simulink model "TBRe19_ECU_1_DAY1_EDIT_190719"  (R2017b)
settings: Solver=FixedStepDiscrete  StartTime=0.0  StopTime=inf  FixedStep=0.0001  RelTol=1e-3
PostLoadFcn:
  | model_init();
libraries: simulink x17
(part 3 of 6)

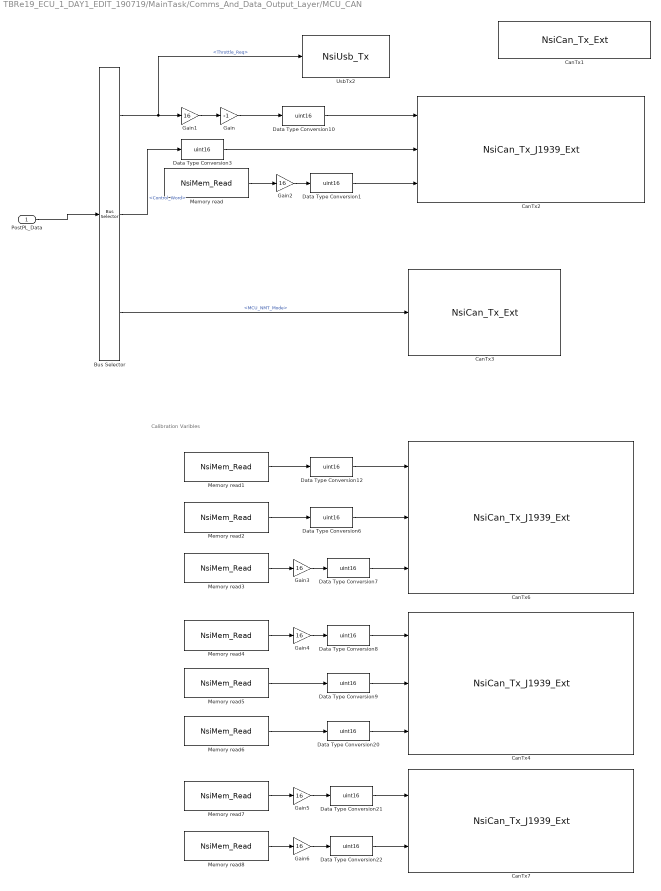
== system TBRe19_ECU_1_DAY1_EDIT_190719/MainTask/Comms_And_Data_Output_Layer/MCU_CAN ==
  note: Calibration Varibles
  PostPL_Data : Inport
  Bus Selector : BusSelector  OutputSignals=VFL_Data.Drive_Data.Throttle_Req,VFL_Data.VOM_Data.Control_Word,VFL_Data.VOM_Data.MCU_NMT_Mode
  CanTx1 : S-Function  FunctionName=NsiCan_Tx_Ext  Parameters=data_can,channel,msg_name,ident,ident_type,dlc,signals,is_physical,is_canfd,is_crc  SFunctionDeploymentMode=off  EnableBusSupport=off  mask(MUXlink Can Tx){data_can=1;HIGH_SPEED;500Kbps;No;C:\Users\TBRe-admin\Documents\Database\TBRe19_DBC_190617.dbc;0;;;0;HIGH_SPEED;500Kbps;120 Ohm;C:\Users\TBRe-admin\Documents\Database\TBRe19_DBC_190517.dbc;0;;;0;HIGH_SPEED;1000Kbps;120 Ohm;D:\TOOLS\MUXLINK\R2011b\MUXlink\misc\BASE_CAN_MUXLAB4.dbc;0;;;0;HIGH_SPEED;500Kbps;120 Ohm;D:\TOOLS\MUXLINK\R2011b\MUXlink\misc\j1939_adapt.dbc;0;;;0;HIGH_SPEED;1000Kbps;No;D:\TOOLS\MUXLINK\R2011b\MUXlink\misc\BASE_CAN_MUXLAB4.dbc;0;;, channel=1, msg_name=MCU_Sync_MSG, ident=0x080, ident_type=STD, dlc=0, signals=, is_physical=0, is_canfd=0, is_crc=0}
      mask prompts: data_can "data can"; msg_name "msg name"
      mask help: Transmit a frame on a CAN Channel.
      mask init:
      | NsiCan_Tx_Ext_InitializationFcn();
      settings: OpenFcn=NsiCan_Tx_Ext_OpenFcn();
      mask Help:
      | eval('block=get_param(gcb, ''RTWdata'');')
      | web([docroot '\toolbox\MUXlink\html\blocks/' block.MUXlink_BlockType '.html'])
      mask Callback data_can: NsiCan_Tx_Ext_ApplyFcn(1);
      mask Callback channel: NsiCan_Tx_Ext_ApplyFcn(2);
      mask Callback msg_name: NsiCan_Tx_Ext_ApplyFcn(3);
      mask Callback ident: NsiCan_Tx_Ext_ApplyFcn(4);
      mask Callback ident_type: NsiCan_Tx_Ext_ApplyFcn(5);
      mask Callback dlc: NsiCan_Tx_Ext_ApplyFcn(6);
      mask Callback signals: NsiCan_Tx_Ext_ApplyFcn(7);
      mask Callback is_physical: NsiCan_Tx_Ext_ApplyFcn(7);
      mask Callback is_canfd: NsiCan_Tx_Ext_ApplyFcn(7);
      mask Callback is_crc: NsiCan_Tx_Ext_ApplyFcn(7);
      mask Display: image(imread('nsi.bmp'));text(0.5, 0.3, 'TX_MCU_Sync_MSG_CAN1', 'horizontalAlignment', 'center', 'verticalAlignment', 'base');plot([0.05 0.05 0.05 0.05 0.05 0.05 0.05 0.05 0.05 0.05]);
  CanTx2 : S-Function  FunctionName=NsiCan_Tx_J1939_Ext  Parameters=data_can,channel,msg_name,ident,ident_type,dlc,signals,is_SA_Masked,is_physical,is_canfd  SFunctionDeploymentMode=off  EnableBusSupport=off  mask(MUXlink Can Tx){data_can=1;HIGH_SPEED;500Kbps;No;C:\Users\Peter\Google_Drive\Year_5\TBRe\03-Design_Files\ECU\ECU-Model\TBRe19_DBC.dbc;0;;;0;HIGH_SPEED;500Kbps;120 Ohm;C:\Users\TBRe-admin\Documents\Database\TBRe19_DBC_190517.dbc;0;;;0;HIGH_SPEED;1000Kbps;120 Ohm;D:\TOOLS\MUXLINK\R2011b\MUXlink\misc\BASE_CAN_MUXLAB4.dbc;0;;;0;HIGH_SPEED;500Kbps;120 Ohm;D:\TOOLS\MUXLINK\R2011b\MUXlink\misc\j1939_adapt.dbc;0;;;0;HIGH_SPEED;1000Kbps;No;D:\TOOLS\MUXLINK\R2011b\MUXlink\misc\BASE_CAN_MUXLAB4.dbc;0;;, channel=1, msg_name=HC1_Demands, ident=0x19107171, ident_type=XTD, dlc=8, signals=Torque_Request;1;0;-16;0.062500;0.000000;Nm;ControlWord;1;16;-16;1.000000;0.000000;_;Torque_Traction_Limit;1;32;-16;0.062500;0.000000;Nm, is_SA_Masked=1, is_physical=0, is_canfd=0}
      mask prompts: data_can "data can"; msg_name "msg name"
      mask help: Transmit a frame on a CAN Channel.
      mask init:
      | NsiCan_Tx_J1939_Ext_InitializationFcn();
      settings: OpenFcn=NsiCan_Tx_J1939_Ext_OpenFcn();
      mask Help:
      | eval('block=get_param(gcb, ''RTWdata'');')
      | web([docroot '\toolbox\MUXlink\html\blocks/' block.MUXlink_BlockType '.html'])
      mask Callback data_can: NsiCan_Tx_J1939_Ext_ApplyFcn(1);
      mask Callback channel: NsiCan_Tx_J1939_Ext_ApplyFcn(2);
      mask Callback msg_name: NsiCan_Tx_J1939_Ext_ApplyFcn(3);
      mask Callback ident: NsiCan_Tx_J1939_Ext_ApplyFcn(4);
      mask Callback ident_type: NsiCan_Tx_J1939_Ext_ApplyFcn(5);
      mask Callback dlc: NsiCan_Tx_J1939_Ext_ApplyFcn(6);
      mask Callback signals: NsiCan_Tx_J1939_Ext_ApplyFcn(7);
      mask Callback is_SA_Masked: NsiCan_Tx_J1939_Ext_ApplyFcn(8);
      mask Callback is_physical: NsiCan_Tx_J1939_Ext_ApplyFcn(9)
      mask Callback is_canfd: NsiCan_Tx_J1939_Ext_ApplyFcn(10)
      mask Display: image(imread('nsi.bmp'));text(0.5, 0.3, 'J1939_PGN  HC1_Demandschannel CAN1', 'horizontalAlignment', 'center', 'verticalAlignment', 'base');plot([0.05 0.05 0.05 0.05 0.05 0.05 0.05 0.05 0.05 0.05]); port_label('input',1, 'Torque_Request'); port_label('input',2, 'ControlWord'); port_label('input',3, 'Torque_Traction_Limit');
  CanTx3 : S-Function  FunctionName=NsiCan_Tx_Ext  Parameters=data_can,channel,msg_name,ident,ident_type,dlc,signals,is_physical,is_canfd,is_crc  SFunctionDeploymentMode=off  EnableBusSupport=off  mask(MUXlink Can Tx){data_can=1;HIGH_SPEED;500Kbps;No;C:\Users\TBRe-admin\Documents\TBReVCU\TBRe19_DBC.dbc;0;;;0;HIGH_SPEED;500Kbps;120 Ohm;C:\Users\TBRe-admin\Documents\Database\TBRe19_DBC_190517.dbc;0;;;0;HIGH_SPEED;1000Kbps;120 Ohm;D:\TOOLS\MUXLINK\R2011b\MUXlink\misc\BASE_CAN_MUXLAB4.dbc;0;;;0;HIGH_SPEED;500Kbps;120 Ohm;D:\TOOLS\MUXLINK\R2011b\MUXlink\misc\j1939_adapt.dbc;0;;;0;HIGH_SPEED;1000Kbps;No;D:\TOOLS\MUXLINK\R2011b\MUXlink\misc\BASE_CAN_MUXLAB4.dbc;0;;, channel=1, msg_name=MCU_NMT_Broadcast, ident=0x070, ident_type=STD, dlc=2, signals=NMT_Command;1;0;8;1.000000;0.000000;_, is_physical=1, is_canfd=0, is_crc=0}
      mask prompts: data_can "data can"; msg_name "msg name"
      mask help: Transmit a frame on a CAN Channel.
      mask init:
      | NsiCan_Tx_Ext_InitializationFcn();
      settings: OpenFcn=NsiCan_Tx_Ext_OpenFcn();
      mask Help:
      | eval('block=get_param(gcb, ''RTWdata'');')
      | web([docroot '\toolbox\MUXlink\html\blocks/' block.MUXlink_BlockType '.html'])
      mask Callback data_can: NsiCan_Tx_Ext_ApplyFcn(1);
      mask Callback channel: NsiCan_Tx_Ext_ApplyFcn(2);
      mask Callback msg_name: NsiCan_Tx_Ext_ApplyFcn(3);
      mask Callback ident: NsiCan_Tx_Ext_ApplyFcn(4);
      mask Callback ident_type: NsiCan_Tx_Ext_ApplyFcn(5);
      mask Callback dlc: NsiCan_Tx_Ext_ApplyFcn(6);
      mask Callback signals: NsiCan_Tx_Ext_ApplyFcn(7);
      mask Callback is_physical: NsiCan_Tx_Ext_ApplyFcn(7);
      mask Callback is_canfd: NsiCan_Tx_Ext_ApplyFcn(7);
      mask Callback is_crc: NsiCan_Tx_Ext_ApplyFcn(7);
      mask Display: image(imread('nsi.bmp'));text(0.5, 0.1, 'TX_MCU_NMT_Broadcast_CAN1', 'horizontalAlignment', 'center', 'verticalAlignment', 'base');plot([0.05 0.05 0.05 0.05 0.05 0.05 0.05 0.05 0.05 0.05]); port_label('input',1, 'NMT_Command');
  CanTx4 : S-Function  FunctionName=NsiCan_Tx_J1939_Ext  Parameters=data_can,channel,msg_name,ident,ident_type,dlc,signals,is_SA_Masked,is_physical,is_canfd  SFunctionDeploymentMode=off  EnableBusSupport=off  mask(MUXlink Can Tx){data_can=1;HIGH_SPEED;500Kbps;No;C:\Users\Peter\Google_Drive\Year_5\TBRe\03-Design_Files\ECU\ECU-Model\TBRe19_DBC.dbc;0;;;0;HIGH_SPEED;500Kbps;120 Ohm;C:\Users\TBRe-admin\Documents\Database\TBRe19_DBC_190517.dbc;0;;;0;HIGH_SPEED;1000Kbps;120 Ohm;D:\TOOLS\MUXLINK\R2011b\MUXlink\misc\BASE_CAN_MUXLAB4.dbc;0;;;0;HIGH_SPEED;500Kbps;120 Ohm;D:\TOOLS\MUXLINK\R2011b\MUXlink\misc\j1939_adapt.dbc;0;;;0;HIGH_SPEED;1000Kbps;No;D:\TOOLS\MUXLINK\R2011b\MUXlink\misc\BASE_CAN_MUXLAB4.dbc;0;;, channel=1, msg_name=HC3_Battery_Demands, ident=0x19127171, ident_type=XTD, dlc=8, signals=DC_Link_Voltage_Target;1;32;-16;0.062500;0.000000;V;DC_Link_Imax_Recharge;1;16;-16;1.000000;0.000000;A;DC_Link_Imax_Discharge;1;0;-16;1.000000;0.000000;A, is_SA_Masked=1, is_physical=0, is_canfd=0}
      mask prompts: data_can "data can"; msg_name "msg name"
      mask help: Transmit a frame on a CAN Channel.
      mask init:
      | NsiCan_Tx_J1939_Ext_InitializationFcn();
      settings: OpenFcn=NsiCan_Tx_J1939_Ext_OpenFcn();
      mask Help:
      | eval('block=get_param(gcb, ''RTWdata'');')
      | web([docroot '\toolbox\MUXlink\html\blocks/' block.MUXlink_BlockType '.html'])
      mask Callback data_can: NsiCan_Tx_J1939_Ext_ApplyFcn(1);
      mask Callback channel: NsiCan_Tx_J1939_Ext_ApplyFcn(2);
      mask Callback msg_name: NsiCan_Tx_J1939_Ext_ApplyFcn(3);
      mask Callback ident: NsiCan_Tx_J1939_Ext_ApplyFcn(4);
      mask Callback ident_type: NsiCan_Tx_J1939_Ext_ApplyFcn(5);
      mask Callback dlc: NsiCan_Tx_J1939_Ext_ApplyFcn(6);
      mask Callback signals: NsiCan_Tx_J1939_Ext_ApplyFcn(7);
      mask Callback is_SA_Masked: NsiCan_Tx_J1939_Ext_ApplyFcn(8);
      mask Callback is_physical: NsiCan_Tx_J1939_Ext_ApplyFcn(9)
      mask Callback is_canfd: NsiCan_Tx_J1939_Ext_ApplyFcn(10)
      mask Display: image(imread('nsi.bmp'));text(0.5, 0.3, 'J1939_PGN  HC3_Battery_Demandschannel CAN1', 'horizontalAlignment', 'center', 'verticalAlignment', 'base');plot([0.05 0.05 0.05 0.05 0.05 0.05 0.05 0.05 0.05 0.05]); port_label('input',1, 'DC_Link_Voltage_Target'); port_label('input',2, 'DC_Link_Imax_Recharge'); port_label('input',3, 'DC_Link_Imax_Discharge');
  CanTx6 : S-Function  FunctionName=NsiCan_Tx_J1939_Ext  Parameters=data_can,channel,msg_name,ident,ident_type,dlc,signals,is_SA_Masked,is_physical,is_canfd  SFunctionDeploymentMode=off  EnableBusSupport=off  mask(MUXlink Can Tx){data_can=1;HIGH_SPEED;500Kbps;No;C:\Users\Peter\Google_Drive\Year_5\TBRe\03-Design_Files\ECU\ECU-Model\TBRe19_DBC.dbc;0;;;0;HIGH_SPEED;500Kbps;120 Ohm;C:\Users\TBRe-admin\Documents\Database\TBRe19_DBC_190517.dbc;0;;;0;HIGH_SPEED;1000Kbps;120 Ohm;D:\TOOLS\MUXLINK\R2011b\MUXlink\misc\BASE_CAN_MUXLAB4.dbc;0;;;0;HIGH_SPEED;500Kbps;120 Ohm;D:\TOOLS\MUXLINK\R2011b\MUXlink\misc\j1939_adapt.dbc;0;;;0;HIGH_SPEED;1000Kbps;No;D:\TOOLS\MUXLINK\R2011b\MUXlink\misc\BASE_CAN_MUXLAB4.dbc;0;;, channel=1, msg_name=HC2_Demands, ident=0x19117171, ident_type=XTD, dlc=8, signals=Speed_Limit_Reverse;1;32;-16;1.000000;0.000000;RPM;Speed_Limit_Forward;1;16;-16;1.000000;0.000000;RPM;Torque_Regen_Limit;1;0;-16;0.062500;0.000000;_, is_SA_Masked=1, is_physical=0, is_canfd=0}
      mask prompts: data_can "data can"; msg_name "msg name"
      mask help: Transmit a frame on a CAN Channel.
      mask init:
      | NsiCan_Tx_J1939_Ext_InitializationFcn();
      settings: OpenFcn=NsiCan_Tx_J1939_Ext_OpenFcn();
      mask Help:
      | eval('block=get_param(gcb, ''RTWdata'');')
      | web([docroot '\toolbox\MUXlink\html\blocks/' block.MUXlink_BlockType '.html'])
      mask Callback data_can: NsiCan_Tx_J1939_Ext_ApplyFcn(1);
      mask Callback channel: NsiCan_Tx_J1939_Ext_ApplyFcn(2);
      mask Callback msg_name: NsiCan_Tx_J1939_Ext_ApplyFcn(3);
      mask Callback ident: NsiCan_Tx_J1939_Ext_ApplyFcn(4);
      mask Callback ident_type: NsiCan_Tx_J1939_Ext_ApplyFcn(5);
      mask Callback dlc: NsiCan_Tx_J1939_Ext_ApplyFcn(6);
      mask Callback signals: NsiCan_Tx_J1939_Ext_ApplyFcn(7);
      mask Callback is_SA_Masked: NsiCan_Tx_J1939_Ext_ApplyFcn(8);
      mask Callback is_physical: NsiCan_Tx_J1939_Ext_ApplyFcn(9)
      mask Callback is_canfd: NsiCan_Tx_J1939_Ext_ApplyFcn(10)
      mask Display: image(imread('nsi.bmp'));text(0.5, 0.3, 'J1939_PGN  HC2_Demandschannel CAN1', 'horizontalAlignment', 'center', 'verticalAlignment', 'base');plot([0.05 0.05 0.05 0.05 0.05 0.05 0.05 0.05 0.05 0.05]); port_label('input',1, 'Speed_Limit_Reverse'); port_label('input',2, 'Speed_Limit_Forward'); port_label('input',3, 'Torque_Regen_Limit');
  CanTx7 : S-Function  FunctionName=NsiCan_Tx_J1939_Ext  Parameters=data_can,channel,msg_name,ident,ident_type,dlc,signals,is_SA_Masked,is_physical,is_canfd  SFunctionDeploymentMode=off  EnableBusSupport=off  mask(MUXlink Can Tx){data_can=1;HIGH_SPEED;500Kbps;No;C:\Users\Peter\Google_Drive\Year_5\TBRe\03-Design_Files\ECU\ECU-Model\TBRe19_DBC.dbc;0;;;0;HIGH_SPEED;500Kbps;120 Ohm;C:\Users\TBRe-admin\Documents\Database\TBRe19_DBC_190517.dbc;0;;;0;HIGH_SPEED;1000Kbps;120 Ohm;D:\TOOLS\MUXLINK\R2011b\MUXlink\misc\BASE_CAN_MUXLAB4.dbc;0;;;0;HIGH_SPEED;500Kbps;120 Ohm;D:\TOOLS\MUXLINK\R2011b\MUXlink\misc\j1939_adapt.dbc;0;;;0;HIGH_SPEED;1000Kbps;No;D:\TOOLS\MUXLINK\R2011b\MUXlink\misc\BASE_CAN_MUXLAB4.dbc;0;;, channel=1, msg_name=HC4_Debug_Demands, ident=0x19137171, ident_type=XTD, dlc=8, signals=Debug_Id_direct_control;1;16;-16;0.062500;0.000000;A;Debug_Iq_direct_control;1;0;-16;0.062500;0.000000;A, is_SA_Masked=1, is_physical=0, is_canfd=0}
      mask prompts: data_can "data can"; msg_name "msg name"
      mask help: Transmit a frame on a CAN Channel.
      mask init:
      | NsiCan_Tx_J1939_Ext_InitializationFcn();
      settings: OpenFcn=NsiCan_Tx_J1939_Ext_OpenFcn();
      mask Help:
      | eval('block=get_param(gcb, ''RTWdata'');')
      | web([docroot '\toolbox\MUXlink\html\blocks/' block.MUXlink_BlockType '.html'])
      mask Callback data_can: NsiCan_Tx_J1939_Ext_ApplyFcn(1);
      mask Callback channel: NsiCan_Tx_J1939_Ext_ApplyFcn(2);
      mask Callback msg_name: NsiCan_Tx_J1939_Ext_ApplyFcn(3);
      mask Callback ident: NsiCan_Tx_J1939_Ext_ApplyFcn(4);
      mask Callback ident_type: NsiCan_Tx_J1939_Ext_ApplyFcn(5);
      mask Callback dlc: NsiCan_Tx_J1939_Ext_ApplyFcn(6);
      mask Callback signals: NsiCan_Tx_J1939_Ext_ApplyFcn(7);
      mask Callback is_SA_Masked: NsiCan_Tx_J1939_Ext_ApplyFcn(8);
      mask Callback is_physical: NsiCan_Tx_J1939_Ext_ApplyFcn(9)
      mask Callback is_canfd: NsiCan_Tx_J1939_Ext_ApplyFcn(10)
      mask Display: image(imread('nsi.bmp'));text(0.5, 0.3, 'J1939_PGN  HC4_Debug_Demandschannel CAN1', 'horizontalAlignment', 'center', 'verticalAlignment', 'base');plot([0.05 0.05 0.05 0.05 0.05 0.05 0.05 0.05 0.05 0.05]); port_label('input',1, 'Debug_Id_direct_control'); port_label('input',2, 'Debug_Iq_direct_control');
  Data Type Conversion{1,3,6..10,12,20..22} (11 alike) : DataTypeConversion  OutDataTypeStr=uint16
  Gain : Gain  Gain=-1  ParamDataTypeStr=int16
  Gain{1..6} (6 alike) : Gain  Gain=16  ParamDataTypeStr=int16
  Memory read : S-Function  FunctionName=NsiMem_Read  Parameters=name_var,type_var,size_var,tunable_var  SFunctionDeploymentMode=off  EnableBusSupport=off  mask(Memory read){name_var=INV_Torque_limit, type_var=Signed Word, size_var=1, tunable_var=on}
      mask prompts: name_var "Variable name :"; type_var "Type :"; size_var "Dim of table :"; tunable_var "Is Tunable By USB?"
      mask help: Reads current value of variable memory declared in the configurator block in calibration page.
      mask init:
      | NsiMem_Read_InitializationFcn();
      settings: OpenFcn=NsiMem_Read_OpenFcn();
      mask Help:
      | eval('block=get_param(gcb, ''RTWdata'');')
      | web([docroot '\toolbox\MUXlink\html\blocks/' block.MUXlink_BlockType '.html'])
      mask TypeOptions name_var: Gearing_Ratio | Wheel_Size | Brake1_High | Brake2_High | Throttle1_High | Throttle2_High | Brake1_Low | Brake2_Low | Throttle1_Low | Throttle2_Low | Max_Torque_Std | Max_Torque_Boost | MCU_Ignition | LV_Low_Voltage_Warning | MCUMotor_Temp_Warning | Target_Slip_Ratio | TC_P_Gain | MinTC_Torque | Max_Regen | Throttle_Active_Threshold | Brake_Active_Threshold | INV_Torque_limit | INV_Speed_Limit_Fwd | INV_Speed_limit_Rev | INV_DC_Link_Target | INV_DC_Link_Regen_Imax | INV_DC_Link_Discharge_Imax | INV_Regen_Torque_Limit | INV_Id_Debug | INV_Iq_debug
      mask Callback name_var: NsiMem_Read_ApplyFcn(1);
      mask TypeOptions type_var: Boolean | Signed Byte | Unsigned Byte | Signed Word | Unsigned Word | Signed Double Word | Unsigned Double Word | Single Float | Double Float
      mask Callback type_var: NsiMem_Read_ApplyFcn(2);
      mask Callback size_var: NsiMem_Read_ApplyFcn(3);
      mask Callback tunable_var: NsiMem_Read_ApplyFcn(4);
      mask Display: image(imread('nsi.bmp'));text(0.5, 0.35, 'INV_Torque_limit', 'horizontalAlignment', 'center', 'verticalAlignment', 'base');plot([0.05 0.05 0.05 0.05 0.05 0.05 0.05 0.05 0.05 0.05]);port_label('output', 1, 'Read');
  Memory read1 : S-Function  FunctionName=NsiMem_Read  Parameters=name_var,type_var,size_var,tunable_var  SFunctionDeploymentMode=off  EnableBusSupport=off  mask(Memory read){name_var=INV_Speed_limit_Rev, type_var=Signed Word, size_var=1, tunable_var=on}
      mask prompts: name_var "Variable name :"; type_var "Type :"; size_var "Dim of table :"; tunable_var "Is Tunable By USB?"
      mask help: Reads current value of variable memory declared in the configurator block in calibration page.
      mask init:
      | NsiMem_Read_InitializationFcn();
      settings: OpenFcn=NsiMem_Read_OpenFcn();
      mask Help:
      | eval('block=get_param(gcb, ''RTWdata'');')
      | web([docroot '\toolbox\MUXlink\html\blocks/' block.MUXlink_BlockType '.html'])
      mask TypeOptions name_var: Gearing_Ratio | Wheel_Size | Brake1_High | Brake2_High | Throttle1_High | Throttle2_High | Brake1_Low | Brake2_Low | Throttle1_Low | Throttle2_Low | Max_Torque_Std | Max_Torque_Boost | MCU_Ignition | LV_Low_Voltage_Warning | MCUMotor_Temp_Warning | Target_Slip_Ratio | TC_P_Gain | MinTC_Torque | Max_Regen | Throttle_Active_Threshold | Brake_Active_Threshold | INV_Torque_limit | INV_Speed_Limit_Fwd | INV_Speed_limit_Rev | INV_DC_Link_Target | INV_DC_Link_Regen_Imax | INV_DC_Link_Discharge_Imax | INV_Regen_Torque_Limit | INV_Id_Debug | INV_Iq_debug
      mask Callback name_var: NsiMem_Read_ApplyFcn(1);
      mask TypeOptions type_var: Boolean | Signed Byte | Unsigned Byte | Signed Word | Unsigned Word | Signed Double Word | Unsigned Double Word | Single Float | Double Float
      mask Callback type_var: NsiMem_Read_ApplyFcn(2);
      mask Callback size_var: NsiMem_Read_ApplyFcn(3);
      mask Callback tunable_var: NsiMem_Read_ApplyFcn(4);
      mask Display: image(imread('nsi.bmp'));text(0.5, 0.35, 'INV_Speed_limit_Rev', 'horizontalAlignment', 'center', 'verticalAlignment', 'base');plot([0.05 0.05 0.05 0.05 0.05 0.05 0.05 0.05 0.05 0.05]);port_label('output', 1, 'Read');
  Memory read2 : S-Function  FunctionName=NsiMem_Read  Parameters=name_var,type_var,size_var,tunable_var  SFunctionDeploymentMode=off  EnableBusSupport=off  mask(Memory read){name_var=INV_Speed_Limit_Fwd, type_var=Signed Word, size_var=1, tunable_var=on}
      mask prompts: name_var "Variable name :"; type_var "Type :"; size_var "Dim of table :"; tunable_var "Is Tunable By USB?"
      mask help: Reads current value of variable memory declared in the configurator block in calibration page.
      mask init:
      | NsiMem_Read_InitializationFcn();
      settings: OpenFcn=NsiMem_Read_OpenFcn();
      mask Help:
      | eval('block=get_param(gcb, ''RTWdata'');')
      | web([docroot '\toolbox\MUXlink\html\blocks/' block.MUXlink_BlockType '.html'])
      mask TypeOptions name_var: Gearing_Ratio | Wheel_Size | Brake1_High | Brake2_High | Throttle1_High | Throttle2_High | Brake1_Low | Brake2_Low | Throttle1_Low | Throttle2_Low | Max_Torque_Std | Max_Torque_Boost | MCU_Ignition | LV_Low_Voltage_Warning | MCUMotor_Temp_Warning | Target_Slip_Ratio | TC_P_Gain | MinTC_Torque | Max_Regen | Throttle_Active_Threshold | Brake_Active_Threshold | INV_Torque_limit | INV_Speed_Limit_Fwd | INV_Speed_limit_Rev | INV_DC_Link_Target | INV_DC_Link_Regen_Imax | INV_DC_Link_Discharge_Imax | INV_Regen_Torque_Limit | INV_Id_Debug | INV_Iq_debug
      mask Callback name_var: NsiMem_Read_ApplyFcn(1);
      mask TypeOptions type_var: Boolean | Signed Byte | Unsigned Byte | Signed Word | Unsigned Word | Signed Double Word | Unsigned Double Word | Single Float | Double Float
      mask Callback type_var: NsiMem_Read_ApplyFcn(2);
      mask Callback size_var: NsiMem_Read_ApplyFcn(3);
      mask Callback tunable_var: NsiMem_Read_ApplyFcn(4);
      mask Display: image(imread('nsi.bmp'));text(0.5, 0.35, 'INV_Speed_Limit_Fwd', 'horizontalAlignment', 'center', 'verticalAlignment', 'base');plot([0.05 0.05 0.05 0.05 0.05 0.05 0.05 0.05 0.05 0.05]);port_label('output', 1, 'Read');
  Memory read3 : S-Function  FunctionName=NsiMem_Read  Parameters=name_var,type_var,size_var,tunable_var  SFunctionDeploymentMode=off  EnableBusSupport=off  mask(Memory read){name_var=INV_Regen_Torque_Limit, type_var=Signed Word, size_var=1, tunable_var=on}
      mask prompts: name_var "Variable name :"; type_var "Type :"; size_var "Dim of table :"; tunable_var "Is Tunable By USB?"
      mask help: Reads current value of variable memory declared in the configurator block in calibration page.
      mask init:
      | NsiMem_Read_InitializationFcn();
      settings: OpenFcn=NsiMem_Read_OpenFcn();
      mask Help:
      | eval('block=get_param(gcb, ''RTWdata'');')
      | web([docroot '\toolbox\MUXlink\html\blocks/' block.MUXlink_BlockType '.html'])
      mask TypeOptions name_var: Gearing_Ratio | Wheel_Size | Brake1_High | Brake2_High | Throttle1_High | Throttle2_High | Brake1_Low | Brake2_Low | Throttle1_Low | Throttle2_Low | Max_Torque_Std | Max_Torque_Boost | MCU_Ignition | LV_Low_Voltage_Warning | MCUMotor_Temp_Warning | Target_Slip_Ratio | TC_P_Gain | MinTC_Torque | Max_Regen | Throttle_Active_Threshold | Brake_Active_Threshold | INV_Torque_limit | INV_Speed_Limit_Fwd | INV_Speed_limit_Rev | INV_DC_Link_Target | INV_DC_Link_Regen_Imax | INV_DC_Link_Discharge_Imax | INV_Regen_Torque_Limit | INV_Id_Debug | INV_Iq_debug
      mask Callback name_var: NsiMem_Read_ApplyFcn(1);
      mask TypeOptions type_var: Boolean | Signed Byte | Unsigned Byte | Signed Word | Unsigned Word | Signed Double Word | Unsigned Double Word | Single Float | Double Float
      mask Callback type_var: NsiMem_Read_ApplyFcn(2);
      mask Callback size_var: NsiMem_Read_ApplyFcn(3);
      mask Callback tunable_var: NsiMem_Read_ApplyFcn(4);
      mask Display: image(imread('nsi.bmp'));text(0.5, 0.35, 'INV_Regen_Torque_Limit', 'horizontalAlignment', 'center', 'verticalAlignment', 'base');plot([0.05 0.05 0.05 0.05 0.05 0.05 0.05 0.05 0.05 0.05]);port_label('output', 1, 'Read');
  Memory read4 : S-Function  FunctionName=NsiMem_Read  Parameters=name_var,type_var,size_var,tunable_var  SFunctionDeploymentMode=off  EnableBusSupport=off  mask(Memory read){name_var=INV_DC_Link_Target, type_var=Signed Word, size_var=1, tunable_var=on}
      mask prompts: name_var "Variable name :"; type_var "Type :"; size_var "Dim of table :"; tunable_var "Is Tunable By USB?"
      mask help: Reads current value of variable memory declared in the configurator block in calibration page.
      mask init:
      | NsiMem_Read_InitializationFcn();
      settings: OpenFcn=NsiMem_Read_OpenFcn();
      mask Help:
      | eval('block=get_param(gcb, ''RTWdata'');')
      | web([docroot '\toolbox\MUXlink\html\blocks/' block.MUXlink_BlockType '.html'])
      mask TypeOptions name_var: Gearing_Ratio | Wheel_Size | Brake1_High | Brake2_High | Throttle1_High | Throttle2_High | Brake1_Low | Brake2_Low | Throttle1_Low | Throttle2_Low | Max_Torque_Std | Max_Torque_Boost | MCU_Ignition | LV_Low_Voltage_Warning | MCUMotor_Temp_Warning | Target_Slip_Ratio | TC_P_Gain | MinTC_Torque | Max_Regen | Throttle_Active_Threshold | Brake_Active_Threshold | INV_Torque_limit | INV_Speed_Limit_Fwd | INV_Speed_limit_Rev | INV_DC_Link_Target | INV_DC_Link_Regen_Imax | INV_DC_Link_Discharge_Imax | INV_Regen_Torque_Limit | INV_Id_Debug | INV_Iq_debug
      mask Callback name_var: NsiMem_Read_ApplyFcn(1);
      mask TypeOptions type_var: Boolean | Signed Byte | Unsigned Byte | Signed Word | Unsigned Word | Signed Double Word | Unsigned Double Word | Single Float | Double Float
      mask Callback type_var: NsiMem_Read_ApplyFcn(2);
      mask Callback size_var: NsiMem_Read_ApplyFcn(3);
      mask Callback tunable_var: NsiMem_Read_ApplyFcn(4);
      mask Display: image(imread('nsi.bmp'));text(0.5, 0.35, 'INV_DC_Link_Target', 'horizontalAlignment', 'center', 'verticalAlignment', 'base');plot([0.05 0.05 0.05 0.05 0.05 0.05 0.05 0.05 0.05 0.05]);port_label('output', 1, 'Read');
  Memory read5 : S-Function  FunctionName=NsiMem_Read  Parameters=name_var,type_var,size_var,tunable_var  SFunctionDeploymentMode=off  EnableBusSupport=off  mask(Memory read){name_var=INV_DC_Link_Regen_Imax, type_var=Signed Word, size_var=1, tunable_var=on}
      mask prompts: name_var "Variable name :"; type_var "Type :"; size_var "Dim of table :"; tunable_var "Is Tunable By USB?"
      mask help: Reads current value of variable memory declared in the configurator block in calibration page.
      mask init:
      | NsiMem_Read_InitializationFcn();
      settings: OpenFcn=NsiMem_Read_OpenFcn();
      mask Help:
      | eval('block=get_param(gcb, ''RTWdata'');')
      | web([docroot '\toolbox\MUXlink\html\blocks/' block.MUXlink_BlockType '.html'])
      mask TypeOptions name_var: Gearing_Ratio | Wheel_Size | Brake1_High | Brake2_High | Throttle1_High | Throttle2_High | Brake1_Low | Brake2_Low | Throttle1_Low | Throttle2_Low | Max_Torque_Std | Max_Torque_Boost | MCU_Ignition | LV_Low_Voltage_Warning | MCUMotor_Temp_Warning | Target_Slip_Ratio | TC_P_Gain | MinTC_Torque | Max_Regen | Throttle_Active_Threshold | Brake_Active_Threshold | INV_Torque_limit | INV_Speed_Limit_Fwd | INV_Speed_limit_Rev | INV_DC_Link_Target | INV_DC_Link_Regen_Imax | INV_DC_Link_Discharge_Imax | INV_Regen_Torque_Limit | INV_Id_Debug | INV_Iq_debug
      mask Callback name_var: NsiMem_Read_ApplyFcn(1);
      mask TypeOptions type_var: Boolean | Signed Byte | Unsigned Byte | Signed Word | Unsigned Word | Signed Double Word | Unsigned Double Word | Single Float | Double Float
      mask Callback type_var: NsiMem_Read_ApplyFcn(2);
      mask Callback size_var: NsiMem_Read_ApplyFcn(3);
      mask Callback tunable_var: NsiMem_Read_ApplyFcn(4);
      mask Display: image(imread('nsi.bmp'));text(0.5, 0.35, 'INV_DC_Link_Regen_Imax', 'horizontalAlignment', 'center', 'verticalAlignment', 'base');plot([0.05 0.05 0.05 0.05 0.05 0.05 0.05 0.05 0.05 0.05]);port_label('output', 1, 'Read');
  Memory read6 : S-Function  FunctionName=NsiMem_Read  Parameters=name_var,type_var,size_var,tunable_var  SFunctionDeploymentMode=off  EnableBusSupport=off  mask(Memory read){name_var=INV_DC_Link_Discharge_Imax, type_var=Signed Word, size_var=1, tunable_var=on}
      mask prompts: name_var "Variable name :"; type_var "Type :"; size_var "Dim of table :"; tunable_var "Is Tunable By USB?"
      mask help: Reads current value of variable memory declared in the configurator block in calibration page.
      mask init:
      | NsiMem_Read_InitializationFcn();
      settings: OpenFcn=NsiMem_Read_OpenFcn();
      mask Help:
      | eval('block=get_param(gcb, ''RTWdata'');')
      | web([docroot '\toolbox\MUXlink\html\blocks/' block.MUXlink_BlockType '.html'])
      mask TypeOptions name_var: Gearing_Ratio | Wheel_Size | Brake1_High | Brake2_High | Throttle1_High | Throttle2_High | Brake1_Low | Brake2_Low | Throttle1_Low | Throttle2_Low | Max_Torque_Std | Max_Torque_Boost | MCU_Ignition | LV_Low_Voltage_Warning | MCUMotor_Temp_Warning | Target_Slip_Ratio | TC_P_Gain | MinTC_Torque | Max_Regen | Throttle_Active_Threshold | Brake_Active_Threshold | INV_Torque_limit | INV_Speed_Limit_Fwd | INV_Speed_limit_Rev | INV_DC_Link_Target | INV_DC_Link_Regen_Imax | INV_DC_Link_Discharge_Imax | INV_Regen_Torque_Limit | INV_Id_Debug | INV_Iq_debug
      mask Callback name_var: NsiMem_Read_ApplyFcn(1);
      mask TypeOptions type_var: Boolean | Signed Byte | Unsigned Byte | Signed Word | Unsigned Word | Signed Double Word | Unsigned Double Word | Single Float | Double Float
      mask Callback type_var: NsiMem_Read_ApplyFcn(2);
      mask Callback size_var: NsiMem_Read_ApplyFcn(3);
      mask Callback tunable_var: NsiMem_Read_ApplyFcn(4);
      mask Display: image(imread('nsi.bmp'));text(0.5, 0.35, 'INV_DC_Link_Discharge_Imax', 'horizontalAlignment', 'center', 'verticalAlignment', 'base');plot([0.05 0.05 0.05 0.05 0.05 0.05 0.05 0.05 0.05 0.05]);port_label('output', 1, 'Read');
  Memory read7 : S-Function  FunctionName=NsiMem_Read  Parameters=name_var,type_var,size_var,tunable_var  SFunctionDeploymentMode=off  EnableBusSupport=off  mask(Memory read){name_var=INV_Id_Debug, type_var=Signed Word, size_var=1, tunable_var=on}
      mask prompts: name_var "Variable name :"; type_var "Type :"; size_var "Dim of table :"; tunable_var "Is Tunable By USB?"
      mask help: Reads current value of variable memory declared in the configurator block in calibration page.
      mask init:
      | NsiMem_Read_InitializationFcn();
      settings: OpenFcn=NsiMem_Read_OpenFcn();
      mask Help:
      | eval('block=get_param(gcb, ''RTWdata'');')
      | web([docroot '\toolbox\MUXlink\html\blocks/' block.MUXlink_BlockType '.html'])
      mask TypeOptions name_var: Gearing_Ratio | Wheel_Size | Brake1_High | Brake2_High | Throttle1_High | Throttle2_High | Brake1_Low | Brake2_Low | Throttle1_Low | Throttle2_Low | Max_Torque_Std | Max_Torque_Boost | MCU_Ignition | LV_Low_Voltage_Warning | MCUMotor_Temp_Warning | Target_Slip_Ratio | TC_P_Gain | MinTC_Torque | Max_Regen | Throttle_Active_Threshold | Brake_Active_Threshold | INV_Torque_limit | INV_Speed_Limit_Fwd | INV_Speed_limit_Rev | INV_DC_Link_Target | INV_DC_Link_Regen_Imax | INV_DC_Link_Discharge_Imax | INV_Regen_Torque_Limit | INV_Id_Debug | INV_Iq_debug
      mask Callback name_var: NsiMem_Read_ApplyFcn(1);
      mask TypeOptions type_var: Boolean | Signed Byte | Unsigned Byte | Signed Word | Unsigned Word | Signed Double Word | Unsigned Double Word | Single Float | Double Float
      mask Callback type_var: NsiMem_Read_ApplyFcn(2);
      mask Callback size_var: NsiMem_Read_ApplyFcn(3);
      mask Callback tunable_var: NsiMem_Read_ApplyFcn(4);
      mask Display: image(imread('nsi.bmp'));text(0.5, 0.35, 'INV_Id_Debug', 'horizontalAlignment', 'center', 'verticalAlignment', 'base');plot([0.05 0.05 0.05 0.05 0.05 0.05 0.05 0.05 0.05 0.05]);port_label('output', 1, 'Read');
  Memory read8 : S-Function  FunctionName=NsiMem_Read  Parameters=name_var,type_var,size_var,tunable_var  SFunctionDeploymentMode=off  EnableBusSupport=off  mask(Memory read){name_var=INV_Iq_debug, type_var=Signed Word, size_var=1, tunable_var=on}
      mask prompts: name_var "Variable name :"; type_var "Type :"; size_var "Dim of table :"; tunable_var "Is Tunable By USB?"
      mask help: Reads current value of variable memory declared in the configurator block in calibration page.
      mask init:
      | NsiMem_Read_InitializationFcn();
      settings: OpenFcn=NsiMem_Read_OpenFcn();
      mask Help:
      | eval('block=get_param(gcb, ''RTWdata'');')
      | web([docroot '\toolbox\MUXlink\html\blocks/' block.MUXlink_BlockType '.html'])
      mask TypeOptions name_var: Gearing_Ratio | Wheel_Size | Brake1_High | Brake2_High | Throttle1_High | Throttle2_High | Brake1_Low | Brake2_Low | Throttle1_Low | Throttle2_Low | Max_Torque_Std | Max_Torque_Boost | MCU_Ignition | LV_Low_Voltage_Warning | MCUMotor_Temp_Warning | Target_Slip_Ratio | TC_P_Gain | MinTC_Torque | Max_Regen | Throttle_Active_Threshold | Brake_Active_Threshold | INV_Torque_limit | INV_Speed_Limit_Fwd | INV_Speed_limit_Rev | INV_DC_Link_Target | INV_DC_Link_Regen_Imax | INV_DC_Link_Discharge_Imax | INV_Regen_Torque_Limit | INV_Id_Debug | INV_Iq_debug
      mask Callback name_var: NsiMem_Read_ApplyFcn(1);
      mask TypeOptions type_var: Boolean | Signed Byte | Unsigned Byte | Signed Word | Unsigned Word | Signed Double Word | Unsigned Double Word | Single Float | Double Float
      mask Callback type_var: NsiMem_Read_ApplyFcn(2);
      mask Callback size_var: NsiMem_Read_ApplyFcn(3);
      mask Callback tunable_var: NsiMem_Read_ApplyFcn(4);
      mask Display: image(imread('nsi.bmp'));text(0.5, 0.35, 'INV_Iq_debug', 'horizontalAlignment', 'center', 'verticalAlignment', 'base');plot([0.05 0.05 0.05 0.05 0.05 0.05 0.05 0.05 0.05 0.05]);port_label('output', 1, 'Read');
  UsbTx2 : S-Function  FunctionName=NsiUsb_Tx  Parameters=signame,resolution,offset,unite  SFunctionDeploymentMode=off  EnableBusSupport=off  mask(MUXlink Usb Tx){signame=TorqueRequestACT, resolution=1, offset=0, unite=Nm}
      mask prompts: signame "Signal name ?"; resolution "Resolution ?"; offset "Offset ?"; unite "Unit ?"
      mask help: Transmit a frame on the USB Channel.
      mask init:
      | NsiUsb_Tx_InitializationFcn();
      settings: OpenFcn=NsiUsb_Tx_OpenFcn();
      mask Help:
      | eval('block=get_param(gcb, ''RTWdata'');')
      | web([docroot '\toolbox\MUXlink\html\blocks/' block.MUXlink_BlockType '.html'])
      mask Callback signame: NsiUsb_Tx_ApplyFcn(1);
      mask Callback resolution: NsiUsb_Tx_ApplyFcn(2);
      mask Callback offset: NsiUsb_Tx_ApplyFcn(3);
      mask Callback unite: NsiUsb_Tx_ApplyFcn(4);
      mask Display: image(imread('nsi.bmp'));text(0.5, 0.2, 'USB Tx', 'horizontalAlignment', 'center', 'verticalAlignment', 'base');plot([0.05 0.05 0.05 0.05 0.05 0.05 0.05 0.05 0.05 0.05]);port_label('input',1, 'TorqueRequestACT');
  wires:
  PostPL_Data/1 -> Bus Selector/1
  Bus Selector/1 -> Gain1/1, UsbTx2/1  "<Throttle_Req>"
  Bus Selector/2 -> Data Type Conversion3/1  "<Control_Word>"
  Bus Selector/3 -> CanTx3/1  "<MCU_NMT_Mode>"
  Data Type Conversion10/1 -> CanTx2/1
  Data Type Conversion3/1 -> CanTx2/2
  Data Type Conversion6/1 -> CanTx6/2
  Data Type Conversion7/1 -> CanTx6/3
  Memory read/1 -> Gain2/1
  Memory read1/1 -> Data Type Conversion12/1
  Data Type Conversion12/1 -> CanTx6/1
  Memory read2/1 -> Data Type Conversion6/1
  Memory read3/1 -> Gain3/1
  Memory read4/1 -> Gain4/1
  Memory read5/1 -> Data Type Conversion9/1
  Memory read6/1 -> Data Type Conversion20/1
  Data Type Conversion8/1 -> CanTx4/1
  Data Type Conversion9/1 -> CanTx4/2
  Data Type Conversion20/1 -> CanTx4/3
  Data Type Conversion21/1 -> CanTx7/1
  Data Type Conversion22/1 -> CanTx7/2
  Memory read7/1 -> Gain5/1
  Memory read8/1 -> Gain6/1
  Data Type Conversion1/1 -> CanTx2/3
  Gain/1 -> Data Type Conversion10/1
  Gain1/1 -> Gain/1
  Gain2/1 -> Data Type Conversion1/1
  Gain3/1 -> Data Type Conversion7/1
  Gain4/1 -> Data Type Conversion8/1
  Gain5/1 -> Data Type Conversion21/1
  Gain6/1 -> Data Type Conversion22/1

== system TBRe19_ECU_1_DAY1_EDIT_190719/MainTask/Post_Processing_Layer/Dash_LEDs ==
  note: Light up RTD button when in RTD mode
  note: Flashes this button LED if LV voltage is low
  VFL_Data : Inport
  Bus Creator : BusCreator  Inputs=5
  Bus Selector : BusSelector  OutputSignals=VOM_Data.Operation_Mode,PrePL_Data.MCU_Temps_Data.MCU_Motor_Temp_Error,PrePL_Data.Pedal_Box_Data.APPS_Implausibility,PrePL_Data.Pedal_Box_Data.APPS_BP_Implausibility,PrePL_Data.LV_Battery.LV_Warning
  Compare To Constant : simulink/Logic and Bit Operations/Compare To Constant  relop===  const=3  OutDataTypeStr=boolean
  Flashy : Stateflow chart  TreatAsAtomicUnit=on
  InitLight : Stateflow chart  TreatAsAtomicUnit=on
  Logical Operator : Logic  Operator=OR  Inputs=3  AllPortsSameDT=off  OutDataTypeStr=boolean
  Logical Operator1 : Logic  AllPortsSameDT=off  OutDataTypeStr=boolean
  Logical Operator{2..5} (4 alike) : Logic  Operator=OR  AllPortsSameDT=off  OutDataTypeStr=boolean
  Wake_Up : Stateflow chart  TreatAsAtomicUnit=on
  LED : Outport
  wires:
  VFL_Data/1 -> Bus Selector/1
  Bus Creator/1 -> LED/1
  Bus Selector/1 -> Compare To Constant/1  "<Operation_Mode>"
  Logical Operator/1 -> Bus Creator/5  "APPS_LED"
  Bus Selector/3 -> Logical Operator/1  "<APPS_Implausibility>"
  InitLight/1(Light) -> Logical Operator/3
  Wake_Up/1(RTD) -> Logical Operator2/1
  Logical Operator2/1 -> Bus Creator/1  "RTD_LED"
  Compare To Constant/1 -> Logical Operator2/2  "btnRTD_LED"
  Logical Operator3/1 -> Bus Creator/2  "X_LED"
  Logical Operator4/1 -> Bus Creator/3  "Y_LED"
  Logical Operator5/1 -> Bus Creator/4  "Z_LED"
  Wake_Up/2(X) -> Logical Operator3/1
  Wake_Up/3(Y) -> Logical Operator4/1
  Wake_Up/4(Z) -> Logical Operator5/1
  Bus Selector/4 -> Logical Operator1/2  "<APPS_BP_Implausibility>"
  Logical Operator1/1 -> Logical Operator/2
  Flashy/1(Light) -> Logical Operator1/1

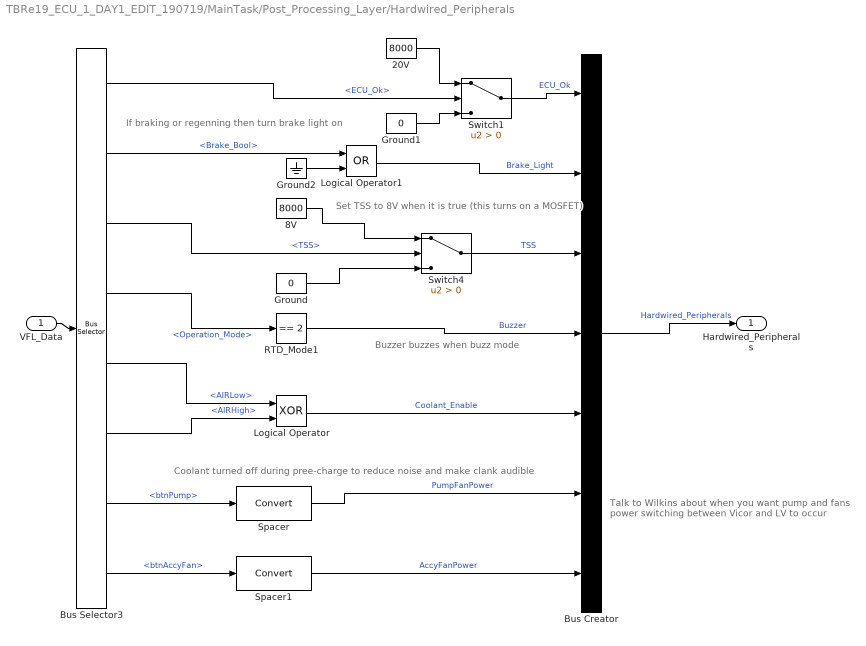
== system TBRe19_ECU_1_DAY1_EDIT_190719/MainTask/Post_Processing_Layer/Hardwired_Peripherals ==
  note: Talk to Wilkins about when you want pump and fans
      | power switching between Vicor and LV to occur
  note: Coolant turned off during pree-charge to reduce noise and make clank audible
  note: Buzzer buzzes when buzz mode
  note: Set TSS to 8V when it is true (this turns on a MOSFET)
  note: If braking or regenning then turn brake light on
  VFL_Data : Inport
  20V : Constant  Value=8000  OutDataTypeStr=Inherit: Inherit via back propagation
  8V : Constant  Value=8000  OutDataTypeStr=Inherit: Inherit via back propagation
  Bus Creator : BusCreator  Inputs=7
  Bus Selector3 : BusSelector  OutputSignals=VOM_Data.ECU_Ok,PrePL_Data.Pedal_Box_Data.Brake_Bool,VOM_Data.TSS,VOM_Data.Operation_Mode,PrePL_Data.DAL_Data.DAL_Hardwired.AIRLow,PrePL_Data.DAL_Data.DAL_Hardwired.AIRHigh,PrePL_Data.Buttons.btnPump,PrePL_Data.Buttons.btnAccyFan
  Ground : Constant  Value=0  OutDataTypeStr=Inherit: Inherit via back propagation
  Ground1 : Constant  Value=0  OutDataTypeStr=Inherit: Inherit via back propagation
  Ground2 : Ground
  Logical Operator : Logic  Operator=XOR  AllPortsSameDT=off  OutDataTypeStr=boolean
  Logical Operator1 : Logic  Operator=OR  AllPortsSameDT=off  OutDataTypeStr=boolean
  RTD_Mode1 : simulink/Logic and Bit Operations/Compare To Constant  relop===  const=2  OutDataTypeStr=boolean
  Spacer : DataTypeConversion
  Spacer1 : DataTypeConversion
  Switch1 : Switch  Criteria=u2 > Threshold  OutDataTypeStr=uint16
  Switch4 : Switch  Criteria=u2 > Threshold  OutDataTypeStr=uint16
  Hardwired_Peripherals : Outport
  wires:
  VFL_Data/1 -> Bus Selector3/1
  Ground/1 -> Switch4/3
  Switch4/1 -> Bus Creator/3  "TSS"
  Bus Selector3/3 -> Switch4/2  "<TSS>"
  8V/1 -> Switch4/1
  Bus Selector3/4 -> RTD_Mode1/1  "<Operation_Mode>"
  Bus Creator/1 -> Hardwired_Peripherals/1  "Hardwired_Peripherals"
  Bus Selector3/2 -> Logical Operator1/1  "<Brake_Bool>"
  Bus Selector3/1 -> Switch1/2  "<ECU_Ok>"
  Logical Operator1/1 -> Bus Creator/2  "Brake_Light"
  RTD_Mode1/1 -> Bus Creator/4  "Buzzer"
  Bus Selector3/5 -> Logical Operator/1  "<AIRLow>"
  Bus Selector3/6 -> Logical Operator/2  "<AIRHigh>"
  Logical Operator/1 -> Bus Creator/5  "Coolant_Enable"
  Bus Selector3/7 -> Spacer/1  "<btnPump>"
  Bus Selector3/8 -> Spacer1/1  "<btnAccyFan>"
  Switch1/1 -> Bus Creator/1  "ECU_Ok"
  20V/1 -> Switch1/1
  Ground1/1 -> Switch1/3
  Ground2/1 -> Logical Operator1/2
  Spacer/1 -> Bus Creator/6  "PumpFanPower"
  Spacer1/1 -> Bus Creator/7  "AccyFanPower"

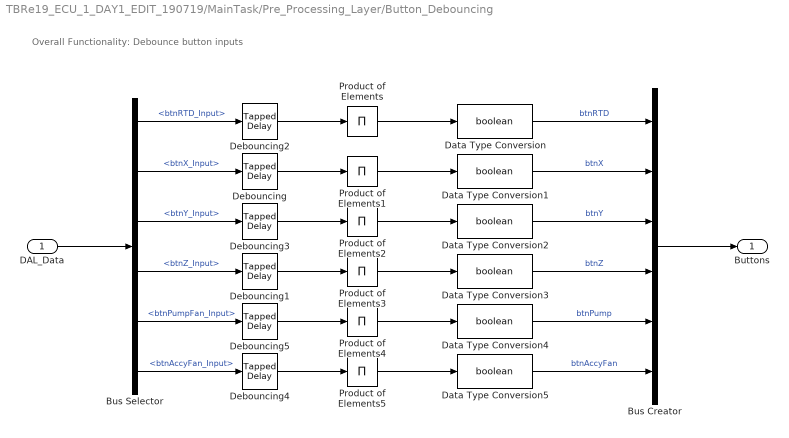
== system TBRe19_ECU_1_DAY1_EDIT_190719/MainTask/Pre_Processing_Layer/Button_Debouncing ==
  note: Overall Functionality:
      | Debounce button inputs
  DAL_Data : Inport
  Bus Creator : BusCreator  Inputs=6
  Bus Selector : BusSelector  OutputSignals=DAL_Hardwired.btnRTD_Input,DAL_Hardwired.btnX_Input,DAL_Hardwired.btnY_Input,DAL_Hardwired.btnZ_Input,DAL_Hardwired.btnPumpFan_Input,DAL_Hardwired.btnAccyFan_Input
  Data Type Conversion{,1..5} (6 alike) : DataTypeConversion  OutDataTypeStr=boolean
  Debouncing{,1..5} (6 alike) : simulink/Discrete/Tapped Delay  vinit=0  samptime=-1  NumDelays=DelayLen  DelayOrder=Oldest  includeCurrent=off
  Product of Elements{,1..5} (6 alike) : Product  Inputs=*
  Buttons : Outport
  wires:
  Product of Elements1/1 -> Data Type Conversion1/1
  Debouncing/1 -> Product of Elements1/1
  Product of Elements/1 -> Data Type Conversion/1
  Debouncing2/1 -> Product of Elements/1
  Bus Selector/2 -> Debouncing/1  "<btnX_Input>"
  DAL_Data/1 -> Bus Selector/1
  Data Type Conversion/1 -> Bus Creator/1  "btnRTD"
  Data Type Conversion1/1 -> Bus Creator/2  "btnX"
  Bus Selector/1 -> Debouncing2/1  "<btnRTD_Input>"
  Bus Creator/1 -> Buttons/1
  Product of Elements2/1 -> Data Type Conversion2/1
  Debouncing3/1 -> Product of Elements2/1
  Debouncing1/1 -> Product of Elements3/1
  Product of Elements3/1 -> Data Type Conversion3/1
  Data Type Conversion2/1 -> Bus Creator/3  "btnY"
  Data Type Conversion3/1 -> Bus Creator/4  "btnZ"
  Bus Selector/3 -> Debouncing3/1  "<btnY_Input>"
  Bus Selector/4 -> Debouncing1/1  "<btnZ_Input>"
  Debouncing5/1 -> Product of Elements4/1
  Debouncing4/1 -> Product of Elements5/1
  Product of Elements4/1 -> Data Type Conversion4/1
  Product of Elements5/1 -> Data Type Conversion5/1
  Bus Selector/5 -> Debouncing5/1  "<btnPumpFan_Input>"
  Bus Selector/6 -> Debouncing4/1  "<btnAccyFan_Input>"
  Data Type Conversion4/1 -> Bus Creator/5  "btnPump"
  Data Type Conversion5/1 -> Bus Creator/6  "btnAccyFan"

== system TBRe19_ECU_1_DAY1_EDIT_190719/MainTask/Pre_Processing_Layer/LV_Battery ==
  note: If voltage is less than or equal to threshold then send CAN
  note: This converts the voltage to a SOC - needs Calibration
  note: This block converts what the ECU thinks the
      | voltage is to what the voltage actually is - Needs Cal
  note: Overall Functionality:
      | To Scale VBAT input and compare to a SOC and a Warning
  DAL_Data : Inport
  Bus Creator : BusCreator  Inputs=3
  Bus Selector : BusSelector  OutputSignals=DAL_Hardwired.LV_Battery_Voltage
  Memory read : S-Function  FunctionName=NsiMem_Read  Parameters=name_var,type_var,size_var,tunable_var  SFunctionDeploymentMode=off  EnableBusSupport=off  mask(Memory read){name_var=LV_Low_Voltage_Warning, type_var=Unsigned Word, size_var=1, tunable_var=on}
      mask prompts: name_var "Variable name :"; type_var "Type :"; size_var "Dim of table :"; tunable_var "Is Tunable By USB?"
      mask help: Reads current value of variable memory declared in the configurator block in calibration page.
      mask init:
      | NsiMem_Read_InitializationFcn();
      settings: OpenFcn=NsiMem_Read_OpenFcn();
      mask Help:
      | eval('block=get_param(gcb, ''RTWdata'');')
      | web([docroot '\toolbox\MUXlink\html\blocks/' block.MUXlink_BlockType '.html'])
      mask TypeOptions name_var: Gearing_Ratio | Wheel_Size | Brake1_High | Brake2_High | Throttle1_High | Throttle2_High | Brake1_Low | Brake2_Low | Throttle1_Low | Throttle2_Low | Max_Torque_Std | Max_Torque_Boost | MCU_Ignition | LV_Low_Voltage_Warning | MCUMotor_Temp_Warning | Target_Slip_Ratio | TC_P_Gain | MinTC_Torque | Max_Regen | Throttle_Active_Threshold | Brake_Active_Threshold | INV_Torque_limit | INV_Speed_Limit_Fwd | INV_Speed_limit_Rev | INV_DC_Link_Target | INV_DC_Link_Regen_Imax | INV_DC_Link_Discharge_Imax | INV_Regen_Torque_Limit | INV_Id_Debug | INV_Iq_debug
      mask Callback name_var: NsiMem_Read_ApplyFcn(1);
      mask TypeOptions type_var: Boolean | Signed Byte | Unsigned Byte | Signed Word | Unsigned Word | Signed Double Word | Unsigned Double Word | Single Float | Double Float
      mask Callback type_var: NsiMem_Read_ApplyFcn(2);
      mask Callback size_var: NsiMem_Read_ApplyFcn(3);
      mask Callback tunable_var: NsiMem_Read_ApplyFcn(4);
      mask Display: image(imread('nsi.bmp'));text(0.5, 0.35, 'LV_Low_Voltage_Warning', 'horizontalAlignment', 'center', 'verticalAlignment', 'base');plot([0.05 0.05 0.05 0.05 0.05 0.05 0.05 0.05 0.05 0.05]);port_label('output', 1, 'Read');
  Relational Operator : RelationalOperator  Operator=<=  OutDataTypeStr=boolean  RndMeth=Simplest
  SOC_Calc : Lookup_n-D  NumberOfTableDimensions=1  BreakpointsForDimension1=[0,16000,24000,24800,25800,26000,26400,33000]  Table=[0,0,10,20,25,50,100,100]  TableDataTypeStr=Inherit: Inherit from 'Table data'  ExtrapMethod=Clip  UseLastTableValue=on  InternalRulePriority=Speed  OutDataTypeStr=uint16  RndMeth=Simplest  InputSameDT=on
  Voltage_Act : Lookup_n-D  NumberOfTableDimensions=1  BreakpointsForDimension1=[0,20000]  Table=[500,33000]  TableDataTypeStr=Inherit: Inherit from 'Table data'  ExtrapMethod=Clip  UseLastTableValue=on  InternalRulePriority=Speed  OutDataTypeStr=uint16  RndMeth=Simplest  InputSameDT=on
  LV_Data : Outport
  wires:
  Bus Creator/1 -> LV_Data/1
  DAL_Data/1 -> Bus Selector/1
  Bus Selector/1 -> Voltage_Act/1  "<LV_Battery_Voltage>"
  Voltage_Act/1 -> Relational Operator/1, Bus Creator/2, SOC_Calc/1  "LV_Battery_Voltage"
  Memory read/1 -> Relational Operator/2
  Relational Operator/1 -> Bus Creator/3  "LV_Warning"
  SOC_Calc/1 -> Bus Creator/1  "LV_SOC%"

== system TBRe19_ECU_1_DAY1_EDIT_190719/MainTask/Pre_Processing_Layer/MCU_Temps ==
  note: Overall Functionality:
      | If either the Motor Temp or the MCU temp is greater than a threshold, then an error is published on the CAN bus
  DAL_Data : Inport
  Bus Creator : BusCreator  Inputs=1
  Bus Selector : BusSelector  OutputSignals=DAL_CAN.DAL_MCUCAN.Motor_Temp,DAL_CAN.DAL_MCUCAN.MCU_Temp
  Memory read : S-Function  FunctionName=NsiMem_Read  Parameters=name_var,type_var,size_var,tunable_var  SFunctionDeploymentMode=off  EnableBusSupport=off  mask(Memory read){name_var=MCUMotor_Temp_Warning, type_var=Unsigned Word, size_var=1, tunable_var=on}
      mask prompts: name_var "Variable name :"; type_var "Type :"; size_var "Dim of table :"; tunable_var "Is Tunable By USB?"
      mask help: Reads current value of variable memory declared in the configurator block in calibration page.
      mask init:
      | NsiMem_Read_InitializationFcn();
      settings: OpenFcn=NsiMem_Read_OpenFcn();
      mask Help:
      | eval('block=get_param(gcb, ''RTWdata'');')
      | web([docroot '\toolbox\MUXlink\html\blocks/' block.MUXlink_BlockType '.html'])
      mask TypeOptions name_var: Gearing_Ratio | Wheel_Size | Brake1_High | Brake2_High | Throttle1_High | Throttle2_High | Brake1_Low | Brake2_Low | Throttle1_Low | Throttle2_Low | Max_Torque_Std | Max_Torque_Boost | MCU_Ignition | LV_Low_Voltage_Warning | MCUMotor_Temp_Warning | Target_Slip_Ratio | TC_P_Gain | MinTC_Torque | Max_Regen | Throttle_Active_Threshold | Brake_Active_Threshold | INV_Torque_limit | INV_Speed_Limit_Fwd | INV_Speed_limit_Rev | INV_DC_Link_Target | INV_DC_Link_Regen_Imax | INV_DC_Link_Discharge_Imax | INV_Regen_Torque_Limit | INV_Id_Debug | INV_Iq_debug
      mask Callback name_var: NsiMem_Read_ApplyFcn(1);
      mask TypeOptions type_var: Boolean | Signed Byte | Unsigned Byte | Signed Word | Unsigned Word | Signed Double Word | Unsigned Double Word | Single Float | Double Float
      mask Callback type_var: NsiMem_Read_ApplyFcn(2);
      mask Callback size_var: NsiMem_Read_ApplyFcn(3);
      mask Callback tunable_var: NsiMem_Read_ApplyFcn(4);
      mask Display: image(imread('nsi.bmp'));text(0.5, 0.35, 'MCUMotor_Temp_Warning', 'horizontalAlignment', 'center', 'verticalAlignment', 'base');plot([0.05 0.05 0.05 0.05 0.05 0.05 0.05 0.05 0.05 0.05]);port_label('output', 1, 'Read');
  MinMax : MinMax  Function=max  Inputs=2
  Relational Operator : RelationalOperator  OutDataTypeStr=boolean  RndMeth=Simplest
  Temp_Data : Outport
  wires:
  Bus Creator/1 -> Temp_Data/1
  DAL_Data/1 -> Bus Selector/1
  Bus Selector/1 -> MinMax/1  "<Motor_Temp>"
  Bus Selector/2 -> MinMax/2  "<MCU_Temp>"
  MinMax/1 -> Relational Operator/1
  Relational Operator/1 -> Bus Creator/1  "MCU_Motor_Temp_Error"
  Memory read/1 -> Relational Operator/2
